simulink model "Junctions9"  (Simulink 8.7)
settings: Solver=FixedStepDiscrete  StartTime=0.0  StopTime=10.0  RelTol=1e-3
settings Model: Creator=sofronis  LastModifiedBy=hamza  ExtModeAutoUpdateStatusClock=off
settings DataIOCC: SignalLoggingSaveFormat=ModelDataLogs  SignalLoggingName=sigsOut
settings DebuggingCC: AlgebraicLoopMsg=error  SaveWithParameterizedLinksMsg=none  SignalResolutionControl=TryResolveAllWithWarning  MultiTaskDSMMsg=warning  MultiTaskCondExecSysMsg=none
settings HardwareCC: TargetUnknown=on
settings SFSimCC: SimParseCustomCode=off
settings GRTTargetCC: GeneratePreprocessorConditionals=Use local settings  CombineOutputUpdateFcns=off  GRTInterface=on

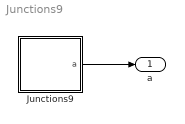
== system Junctions9 ==
  Junctions9 : Stateflow chart  TreatAsAtomicUnit=on
  a : Outport
  wires:
  Junctions9/1(a) -> a/1

== stateflow chart Junctions9 ==
  state A
  state C
  state B
  (junction 9) -> B : [myfalse] {a+=100}
  (default) -> A : {a = 0}
  (junction 10) -> (junction 9) [order 1] : [mytrue] {a+=10}
  A -> (junction 10) : [mytrue] {a+=1}
  (junction 10) -> C [order 2] : [mytrue] {a+=1000}
  data: mytrue constant boolean =1; myfalse constant boolean; a output double
